simulink model "CAPSM_IEEE39_260305_113304"  (R2025b)
settings: Solver=ode45  StartTime=0  StopTime=100  MaxStep=0.001  RelTol=1e-3  AbsTol=1e-4
settings Model: Creator=mtk17  LastModifiedBy=mtk17

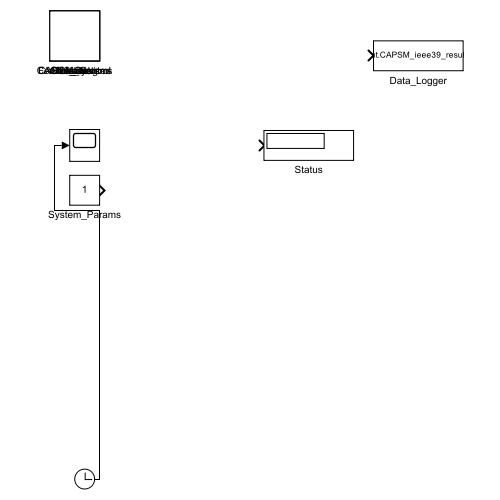
[thumbnail: Simulink's stored preview of the top-level diagram]
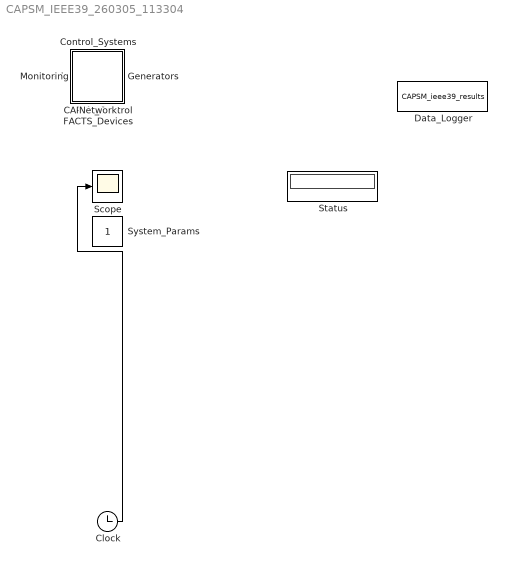
== system CAPSM_IEEE39_260305_113304 ==
  CAPSM_Control : Subsystem
  Clock : Clock
  Control_Systems : Subsystem
  Data_Logger : ToWorkspace  VariableName=CAPSM_ieee39_results  SaveFormat=Timeseries  SampleTime=-1
  FACTS_Devices : Subsystem
  Generators : Subsystem
  Loads : Subsystem
  Monitoring : Subsystem
  Network : Subsystem
  Scope : Scope
  Status : Display
  System_Params : Constant
  wires:
  Clock/1 -> Scope/1

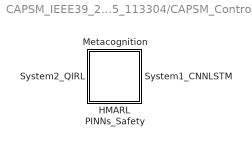
== system CAPSM_IEEE39_260305_113304/CAPSM_Control ==
  HMARL : Subsystem
  Metacognition : Subsystem
  PINNs_Safety : Subsystem
  System1_CNNLSTM : Subsystem
  System2_QIRL : Subsystem

== system CAPSM_IEEE39_260305_113304/Control_Systems ==

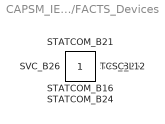
== system CAPSM_IEEE39_260305_113304/FACTS_Devices ==
  STATCOM_B16 : Constant
  STATCOM_B21 : Constant
  STATCOM_B24 : Constant
  SVC_B25 : Constant
  SVC_B26 : Constant
  TCSC_L12 : Constant

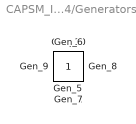
== system CAPSM_IEEE39_260305_113304/Generators ==
  Gen_{1..10} (10 alike) : Constant

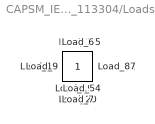
== system CAPSM_IEEE39_260305_113304/Loads ==
  Load_{1..20} (20 alike) : Constant

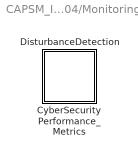
== system CAPSM_IEEE39_260305_113304/Monitoring ==
  CyberSecurity : Subsystem
  DisturbanceDetection : Subsystem
  Performance_Metrics : Subsystem

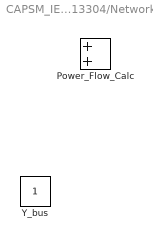
== system CAPSM_IEEE39_260305_113304/Network ==
  Power_Flow_Calc : Sum
  Y_bus : Constant

== system CAPSM_IEEE39_260305_113304/CAPSM_Control/HMARL ==

== system CAPSM_IEEE39_260305_113304/CAPSM_Control/Metacognition ==

== system CAPSM_IEEE39_260305_113304/CAPSM_Control/PINNs_Safety ==

== system CAPSM_IEEE39_260305_113304/CAPSM_Control/System1_CNNLSTM ==

== system CAPSM_IEEE39_260305_113304/CAPSM_Control/System2_QIRL ==

== system CAPSM_IEEE39_260305_113304/Monitoring/CyberSecurity ==

== system CAPSM_IEEE39_260305_113304/Monitoring/DisturbanceDetection ==

== system CAPSM_IEEE39_260305_113304/Monitoring/Performance_Metrics ==
